simulink model "sigmadelta_csett_to_PDM"  (Simulink 7.4)
settings: Solver=ode45  StartTime=0.0  StopTime=10000.0  RelTol=1e-3
settings Model: Creator=Tibor  LastModifiedBy=Tibor

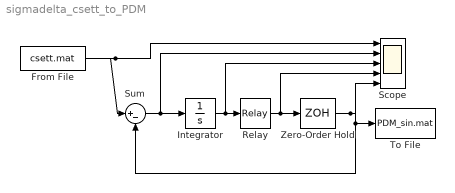
== system sigmadelta_csett_to_PDM ==
  From File : FromFile  FileName=csett.mat  SampleTime=0
  Integrator : Integrator
  Relay : Relay  OnSwitchValue=0  OffSwitchValue=0  OffOutputValue=-1  OutDataType=fixdt(1, 16)  OutScaling=2^0
  Scope : Scope  NumInputPorts=5
      settings: YMin=-5~-5~-5~-5~-5  YMax=5~5~5~5~5  SampleInput=on
  Sum : Sum  Inputs=|+-  OutDataType=fixdt(1, 16)  OutScaling=2^0
  To File : ToFile  Filename=PDM_sin.mat
  Zero-Order Hold : ZeroOrderHold
  wires:
  Sum/1 -> Integrator/1, Scope/2
  Integrator/1 -> Relay/1, Scope/3
  Zero-Order Hold/1 -> Scope/5, Sum/2, To File/1
  Relay/1 -> Zero-Order Hold/1, Scope/4
  From File/1 -> Scope/1, Sum/1
